simulink model "PV"  (R2018b)
settings: Solver=VariableStepAuto  StartTime=0.0  StopTime=10.0  RelTol=1e-3
undefined symbols (not defined in the file or in its folder): Pv
settings Model: Creator=Pedro  LastModifiedBy=Pedro

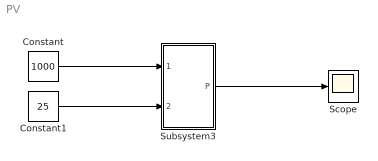
== system PV ==
  Constant : Constant  Value=1000
  Constant1 : Constant  Value=25
  Scope : Scope
  Subsystem3 : Subsystem
  wires:
  Constant/1 -> Subsystem3/1(PvF_Irra)
  Constant1/1 -> Subsystem3/2(PvF_Tamb)
  Subsystem3/1(P) -> Scope/1

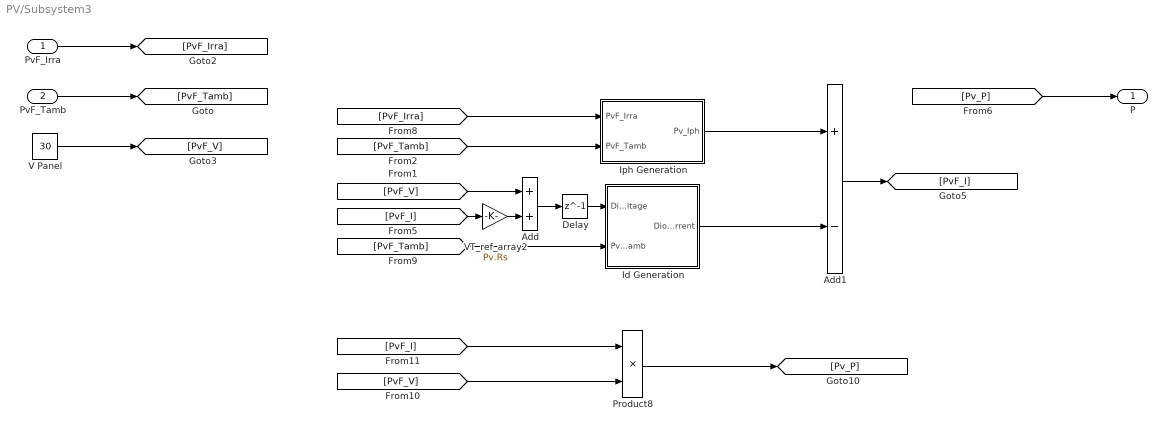
== system PV/Subsystem3 ==
  PvF_Irra : Inport
  PvF_Tamb : Inport  Port=2
  Add : Sum
  Add1 : Sum  Inputs=+-
  Delay : Delay  DelayLength=1
  Id Generation : Subsystem
  Iph Generation : Subsystem
  Product8 : Product  Inputs=**  RndMeth=Zero
  V Panel : Constant  Value=30
  VT_ref_array2 : Gain  Gain=Pv.Rs
  P : Outport
  wires:
  Delay/1 -> Id Generation/1(Diode Voltage)
  Iph Generation/1(Pv_Iph) -> Add1/1
  Add1/1 -> [PvF_I]
  PvF_Tamb/1 -> [PvF_Tamb]
  PvF_Irra/1 -> [PvF_Irra]
  Add/1 -> Delay/1
  Id Generation/1(Diode Current) -> Add1/2
  V Panel/1 -> [PvF_V]
  VT_ref_array2/1 -> Add/2
  Product8/1 -> [Pv_P]
  [PvF_V] -> Product8/2
  [PvF_I] -> Product8/1
  [PvF_I] -> VT_ref_array2/1
  [Pv_P] -> P/1
  [PvF_V] -> Add/1
  [PvF_Tamb] -> Id Generation/2(PvF_Tamb)
  [PvF_Tamb] -> Iph Generation/2(PvF_Tamb)
  [PvF_Irra] -> Iph Generation/1(PvF_Irra)

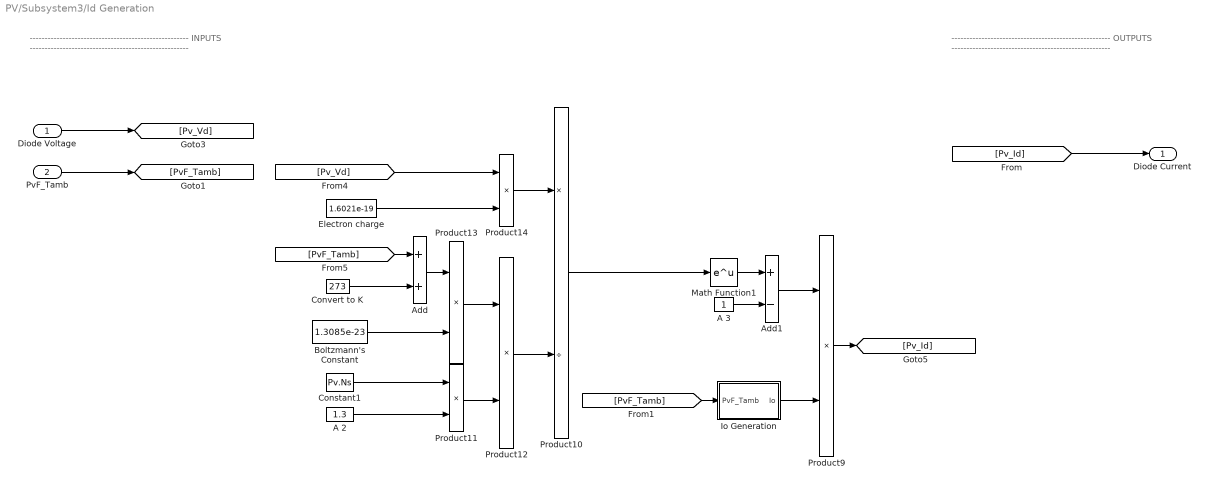
== system PV/Subsystem3/Id Generation ==
  note: -----------------------------------------------------
      |                          INPUTS
      | -----------------------------------------------------
  note: -----------------------------------------------------
      |                          OUTPUTS
      | -----------------------------------------------------
  Diode Voltage : Inport
  PvF_Tamb : Inport  Port=2
  A 2 : Constant  Value=1.3
  A 3 : Constant
  Add : Sum
  Add1 : Sum  Inputs=+-
  "Boltzmann's Constant " : Constant  Value=1.3085e-23
  Constant1 : Constant  Value=Pv.Ns
  Convert to K : Constant  Value=273
  Electron charge : Constant  Value=1.6021e-19
  Io Generation : Subsystem
  Math Function1 : Math  SaturateOnIntegerOverflow=on
  Product10 : Product  Inputs=*/  RndMeth=Zero
  Product{9,11..14} (5 alike) : Product  Inputs=**  RndMeth=Zero
  Diode Current : Outport
  wires:
  Constant1/1 -> Product11/1
  [PvF_Tamb] -> Io Generation/1(PvF_Tamb)
  "Boltzmann's Constant "/1 -> Product13/2
  Product10/1 -> Math Function1/1
  Add/1 -> Product13/1
  Add1/1 -> Product9/1
  A 3/1 -> Add1/2
  Electron charge/1 -> Product14/2
  Product12/1 -> Product10/2
  A 2/1 -> Product11/2
  Io Generation/1(Io) -> Product9/2
  Product14/1 -> Product10/1
  Product13/1 -> Product12/1
  Product11/1 -> Product12/2
  Convert to K/1 -> Add/2
  Math Function1/1 -> Add1/1
  Product9/1 -> [Pv_Id]
  Diode Voltage/1 -> [Pv_Vd]
  [PvF_Tamb] -> Add/1
  PvF_Tamb/1 -> [PvF_Tamb]
  [Pv_Vd] -> Product14/1
  [Pv_Id] -> Diode Current/1

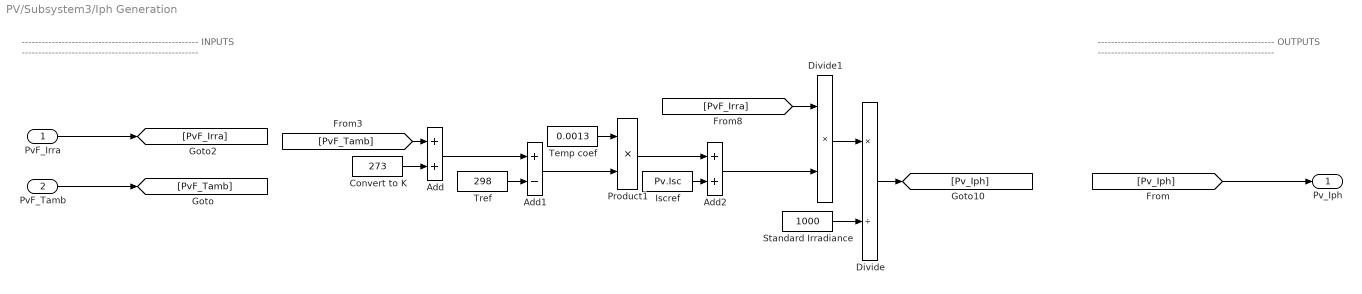
== system PV/Subsystem3/Iph Generation ==
  note: -----------------------------------------------------
      |                          INPUTS
      | -----------------------------------------------------
  note: -----------------------------------------------------
      |                          OUTPUTS
      | -----------------------------------------------------
  PvF_Irra : Inport
  PvF_Tamb : Inport  Port=2
  Add : Sum
  Add1 : Sum  Inputs=+-
  Add2 : Sum
  "Convert to K " : Constant  Value=273
  Divide : Product  Inputs=*/
  Divide1 : Product  Inputs=**
  Iscref : Constant  Value=Pv.Isc
  Product1 : Product
  Standard Irradiance : Constant  Value=1000
  Temp coef : Constant  Value=0.0013
  "Tref " : Constant  Value=298
  Pv_Iph : Outport
  wires:
  Divide1/1 -> Divide/1
  Divide/1 -> [Pv_Iph]
  Temp coef/1 -> Product1/1
  Product1/1 -> Add2/1
  Standard Irradiance/1 -> Divide/2
  Add/1 -> Add1/1
  Add1/1 -> Product1/2
  [PvF_Tamb] -> Add/1
  [Pv_Iph] -> Pv_Iph/1
  PvF_Tamb/1 -> [PvF_Tamb]
  PvF_Irra/1 -> [PvF_Irra]
  "Convert to K "/1 -> Add/2
  "Tref "/1 -> Add1/2
  Iscref/1 -> Add2/2
  Add2/1 -> Divide1/2
  [PvF_Irra] -> Divide1/1

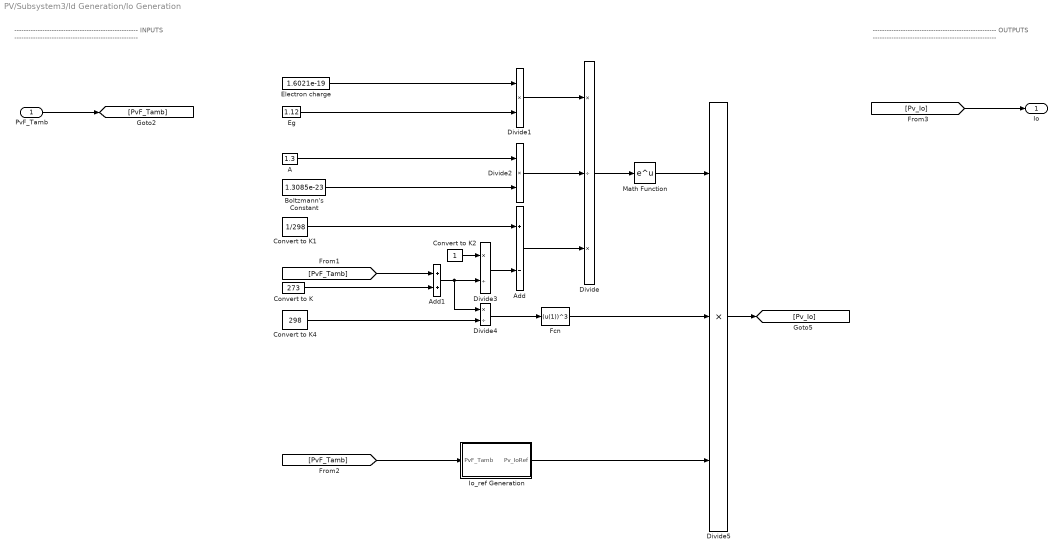
== system PV/Subsystem3/Id Generation/Io Generation ==
  note: -----------------------------------------------------
      |                          INPUTS
      | -----------------------------------------------------
  note: -----------------------------------------------------
      |                          OUTPUTS
      | -----------------------------------------------------
  PvF_Tamb : Inport
  "A " : Constant  Value=1.3
  Add : Sum  Inputs=+-
  Add1 : Sum
  Boltzmann's Constant : Constant  Value=1.3085e-23
  Convert to K : Constant  Value=273
  Convert to K1 : Constant  Value=1/298
  Convert to K2 : Constant
  Convert to K4 : Constant  Value=298
  Divide : Product  Inputs=*/*
  Divide1 : Product  Inputs=**
  Divide2 : Product  Inputs=**
  Divide3 : Product  Inputs=*/
  Divide4 : Product  Inputs=*/
  Divide5 : Product  Inputs=***
  Eg : Constant  Value=1.12
  Electron charge : Constant  Value=1.6021e-19
  Fcn : Fcn  Expr=(u(1))^3
  Io_ref Generation : Subsystem
  Math Function : Math  SaturateOnIntegerOverflow=on
  Io : Outport
  wires:
  PvF_Tamb/1 -> [PvF_Tamb]
  Add1/1 -> Divide4/1, Divide3/2
  [PvF_Tamb] -> Add1/1
  Convert to K/1 -> Add1/2
  Electron charge/1 -> Divide1/1
  Eg/1 -> Divide1/2
  Divide1/1 -> Divide/1
  "A "/1 -> Divide2/1
  Boltzmann's Constant/1 -> Divide2/2
  Divide2/1 -> Divide/2
  Convert to K1/1 -> Add/1
  Add/1 -> Divide/3
  Convert to K2/1 -> Divide3/1
  Divide3/1 -> Add/2
  Convert to K4/1 -> Divide4/2
  Divide4/1 -> Fcn/1
  Fcn/1 -> Divide5/2
  Io_ref Generation/1(Pv_IoRef) -> Divide5/3
  Divide/1 -> Math Function/1
  Math Function/1 -> Divide5/1
  Divide5/1 -> [Pv_Io]
  [Pv_Io] -> Io/1
  [PvF_Tamb] -> Io_ref Generation/1(PvF_Tamb)

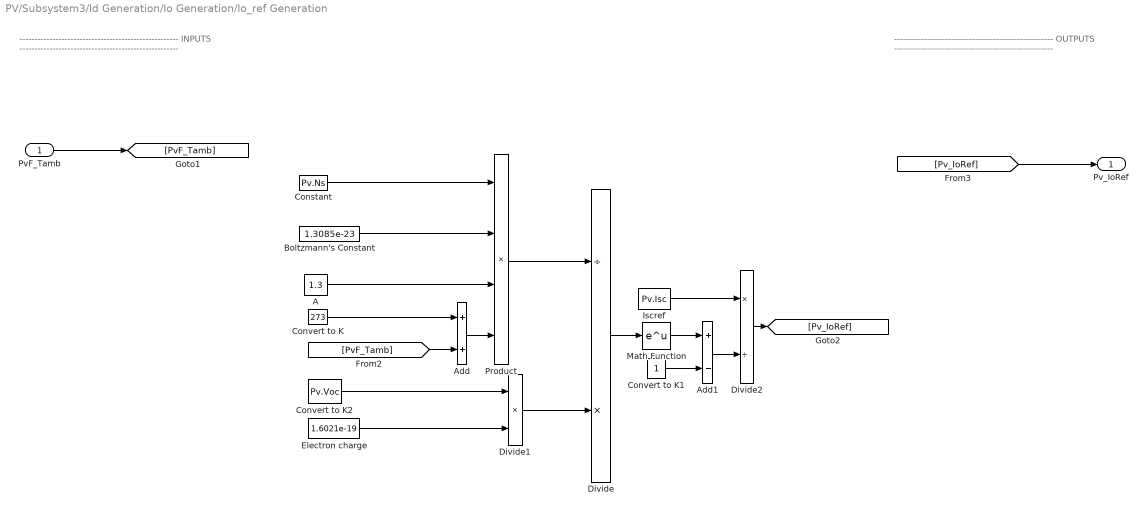
== system PV/Subsystem3/Id Generation/Io Generation/Io_ref Generation ==
  note: -----------------------------------------------------
      |                          INPUTS
      | -----------------------------------------------------
  note: -----------------------------------------------------
      |                          OUTPUTS
      | -----------------------------------------------------
  PvF_Tamb : Inport
  "A " : Constant  Value=1.3
  Add : Sum
  Add1 : Sum  Inputs=+-
  Boltzmann's Constant : Constant  Value=1.3085e-23
  Constant : Constant  Value=Pv.Ns
  Convert to K : Constant  Value=273
  Convert to K1 : Constant
  Convert to K2 : Constant  Value=Pv.Voc
  Divide : Product  Inputs=/*
  Divide1 : Product  Inputs=**
  Divide2 : Product  Inputs=*/
  Electron charge : Constant  Value=1.6021e-19
  Iscref : Constant  Value=Pv.Isc
  Math Function : Math  SaturateOnIntegerOverflow=on
  Product : Product  Inputs=4
  Pv_IoRef : Outport
  wires:
  PvF_Tamb/1 -> [PvF_Tamb]
  Divide2/1 -> [Pv_IoRef]
  [Pv_IoRef] -> Pv_IoRef/1
  Constant/1 -> Product/1
  Boltzmann's Constant/1 -> Product/2
  "A "/1 -> Product/3
  Convert to K/1 -> Add/1
  Product/1 -> Divide/1
  Divide/1 -> Math Function/1
  Math Function/1 -> Add1/1
  Add1/1 -> Divide2/2
  Iscref/1 -> Divide2/1
  Divide1/1 -> Divide/2
  Electron charge/1 -> Divide1/2
  Convert to K2/1 -> Divide1/1
  [PvF_Tamb] -> Add/2
  Add/1 -> Product/4
  Convert to K1/1 -> Add1/2
